simulink subsystem "yarn_model"  (R2023b)
settings: Solver=VariableStepAuto  StartTime=0.0  StopTime=10.0  RelTol=1e-3
values from neighbouring files (symbols this model uses):
  res_mdl_params =     [mdl_parameters_int.mat]
libraries: cstblocks x1
settings Model: Creator=Previ  LastModifiedBy=Previ

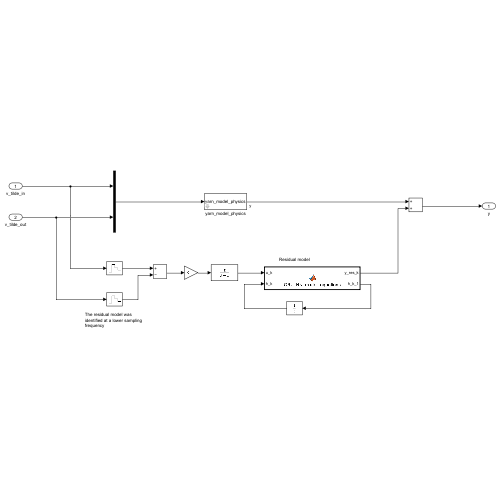
[thumbnail: Simulink's stored preview of the top-level diagram]
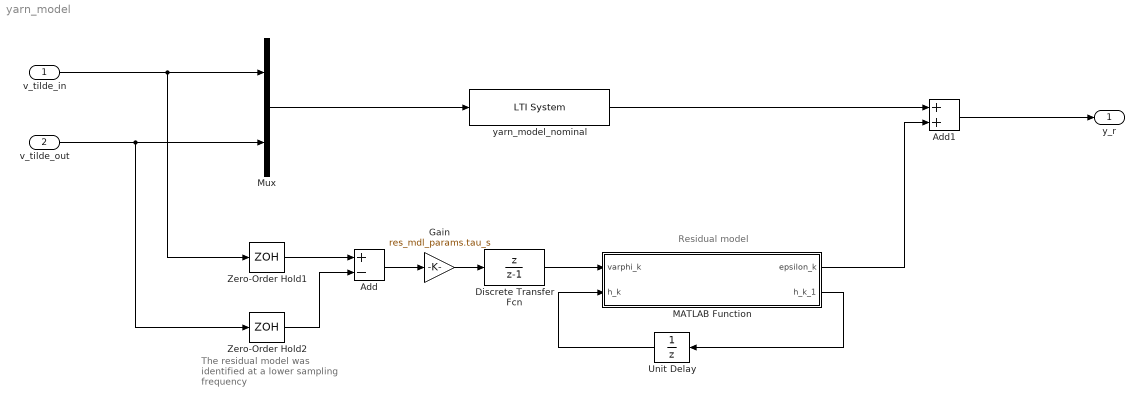
== system yarn_model ==
  note: The residual model was identified at a lower sampling frequency
  note: Residual model
  v_tilde_in : Inport  PortDimensions=[1, 1]
  v_tilde_out : Inport  Port=2  PortDimensions=[1, 1]
  Add : Sum  Inputs=+-
  Add1 : Sum
  Discrete Transfer Fcn : DiscreteTransferFcn  Numerator=[1 0]  Denominator=[1 -1]
  Gain : Gain  Gain=res_mdl_params.tau_s
  MATLAB Function : MATLAB Function  TreatAsAtomicUnit=on
  Mux : Mux  Inputs=2
  Unit Delay : UnitDelay  SampleTime=res_mdl_params.tau_s  HasFrameUpgradeWarning=on
  Zero-Order Hold1 : ZeroOrderHold  SampleTime=res_mdl_params.tau_s
  Zero-Order Hold2 : ZeroOrderHold  SampleTime=res_mdl_params.tau_s
  yarn_model_nominal : cstblocks/LTI System  sys=yarn_model_nominal  IC=0  PadeOrder=0
  y_r : Outport  PortDimensions=[1, 1]
  wires:
  Zero-Order Hold2/1 -> Add/2
  yarn_model_nominal/1 -> Add1/1
  Zero-Order Hold1/1 -> Add/1
  Discrete Transfer Fcn/1 -> MATLAB Function/1(varphi_k)
  MATLAB Function/2(h_k_1) -> Unit Delay/1
  Add/1 -> Gain/1
  v_tilde_out/1 -> Zero-Order Hold2/1, Mux/2
  Gain/1 -> Discrete Transfer Fcn/1
  v_tilde_in/1 -> Zero-Order Hold1/1, Mux/1
  Unit Delay/1 -> MATLAB Function/2(h_k)
  Mux/1 -> yarn_model_nominal/1
  Add1/1 -> y_r/1
  MATLAB Function/1(epsilon_k) -> Add1/2

== matlab function yarn_model/MATLAB Function ==
  data: varphi_k input size=[1, 1]; h_k input size=[res_mdl_params.n_h_tot, 1]; epsilon_k output size=[1, 1]; h_k_1 output size=[res_mdl_params.n_h_tot, 1]; res_mdl_params parameter
function [epsilon_k, h_k_1] = GRU_NN_model_equations(varphi_k, h_k, res_mdl_params)
start_idx = nan(1, 1);
end_idx = nan(1, 1);

% Standardize input
varphi_k = (varphi_k - res_mdl_params.varphi_mean)./res_mdl_params.varphi_std;

% Divide into hidden layers
h_k_1 = nan(size(h_k));
for j = 1 : res_mdl_params.N_layers
    if j > 1
        varphi_k = h_k_1(start_idx : end_idx);
    end

    start_idx = sum(res_mdl_params.n_h(1 : j - 1)) + 1;
    end_idx = sum(res_mdl_params.n_h(1 : j));
    h_k_l = h_k(start_idx : end_idx);

    % Unpad weights and biases
    W_r = res_mdl_params.W(j).W_r(1 : res_mdl_params.W_height(j), 1 : res_mdl_params.W_width(j));
    W_z = res_mdl_params.W(j).W_z(1 : res_mdl_params.W_height(j), 1 : res_mdl_params.W_width(j));
    W_h = res_mdl_params.W(j).W_h(1 : res_mdl_params.W_height(j), 1 : res_mdl_params.W_width(j));
    R_r = res_mdl_params.R(j).R_r(1 : res_mdl_params.R_height(j), 1 : res_mdl_params.R_width(j));
    R_z = res_mdl_params.R(j).R_z(1 : res_mdl_params.R_height(j), 1 : res_mdl_params.R_width(j));
    R_h = res_mdl_params.R(j).R_h(1 : res_mdl_params.R_height(j), 1 : res_mdl_params.R_width(j));
    b_r = res_mdl_params.b(j).b_r(1 : res_mdl_params.b_height(j), 1 : res_mdl_params.b_width(j));
    b_z = res_mdl_params.b(j).b_z(1 : res_mdl_params.b_height(j), 1 : res_mdl_params.b_width(j));
    b_h = res_mdl_params.b(j).b_h(1 : res_mdl_params.b_height(j), 1 : res_mdl_params.b_width(j));

    % Compute gates
    r_k = sigmoid_f(W_r * varphi_k + R_r * h_k_l + b_r);
    z_k = sigmoid_f(W_z * varphi_k + R_z * h_k_l + b_z);
    h_tilde_k = tanh_f(W_h * varphi_k + r_k .* (R_h * h_k_l) + b_h);

    % Compute state update
    h_k_1(start_idx : end_idx) = (1 - z_k) .* h_tilde_k + z_k .* h_k_l;
end

% Compute feedforward mapping
epsilon_k = res_mdl_params.W_FF * h_k_1(start_idx : end_idx) + res_mdl_params.b_FF;

% De-standardize output
epsilon_k = (epsilon_k * res_mdl_params.epsilon_std) + res_mdl_params.epsilon_mean;
end

% Component-wise Sigmoid function
function out = sigmoid_f(in)
out = 1 ./ (1 + exp(-in));
end

% Component-wise Hyperbolic Tangent (tanh) function
function out = tanh_f(in)
out = (exp(in) - exp(-in)) ./ (exp(in) + exp(-in));
end
